simulink model "Ford_T3T6_ArchCnctnDigrm"  (R2016b)
settings: Solver=FixedStepDiscrete  StartTime=0.0  StopTime=10.0  RelTol=1e-3  EnableMultiTasking=on
libraries: canmsglib x15
(part 3 of 15)

== system Ford_T3T6_ArchCnctnDigrm/States and Modes ==
  note: Use Ground if we are using only Gate drive 0 control
  note: T3 does not use SF061
      | (SteerMod)
  note: ASIL D
  note: ASIL D
  note: ASIL D
  note: NM001
  note: NM001
  note: ASIL D
  ES002A_McuDiagc : Subsystem  Tag=3.0.1  Description=This FDD contains uCDiagnostics that are implemented purely with software and are not dependent upon electrical architecture.
      settings: AttributesFormatString=Version: %<Tag>
  ES100A_SysStMod : Subsystem  Tag=1.3.0  Description=Controls the operating state of the system
      settings: AttributesFormatString=Version: %<Tag>
  Ground : Ground
  SF048A_TqLoa : Subsystem  Tag=1.4.1  Description=This function provides a position-based assist command. It also outputs a validity flag to indicate if the TrqLOACmd is valid.
      settings: AttributesFormatString=Version: %<Tag>
  SF049B_LoaMgr : Subsystem  Tag=1.0.0  Description="This function monitors monitors sensor redundancy and allows the choice of system response to varying numbers and types of sensors being unavailable.  It outputs operating state information that other functions use to modify their own behavior when appropriate.  It also outputs a desired system scale factor and slew rate, arbitrated in SF005A State Output Control and then applied in SF004B Assist Sum and Limit."
      settings: AttributesFormatString=Version: %<Tag>
  SystemStartUpState : Subsystem
  tag scope: HwTqLoaMtgtnEna=global, LoaRateLim=global, LoaSca=global, LoaSt=global, LoopCntr2MilliSec=global, MotAgLoaMtgtnEna=global, MotAndThermProtnLoaMod=global, MotCtrlFastLoopCntr=global, MotCtrlSlowLoopCntr=global, SysSt=global, TqLoaAvl=global, TqLoaCmd=global
  wires:
  ES100A_SysStMod/1(SysSt) -> SystemStartUpState/1(SysSt), [SysSt]
  SystemStartUpState/1(SysStWrmIninCmpl) -> ES100A_SysStMod/6(SysStWrmIninCmpl)
  SystemStartUpState/2(StrtUpSt) -> ES100A_SysStMod/7(StrtUpSt)
  [SysStFltOutpReqDi] -> ES100A_SysStMod/2(SysStFltOutpReqDi)
  [SysStImdtTranReqOff] -> ES100A_SysStMod/3(SysStImdtTranReqOff)
  [SysStReqDi] -> ES100A_SysStMod/4(SysStReqDi)
  [FordSysStReqEna] -> ES100A_SysStMod/5(SysStReqEna)
  [FordPwrSplyEnaReq] -> ES100A_SysStMod/1(PwrSplyEnaReq)
  [CurrMeasIdptSig] -> SF049B_LoaMgr/1(CurrMeasIdptSig)
  [DiagcStsIvtr1Inactv] -> SF049B_LoaMgr/2(DiagcStsIvtr1Inactv)
  [DiagcStsIvtr2Inactv] -> SF049B_LoaMgr/3(DiagcStsIvtr2Inactv)
  [HwTqIdptSig] -> SF049B_LoaMgr/4(HwTqIdptSig)
  [IvtrFetFltTyp] -> SF049B_LoaMgr/5(IvtrFetFltTyp)
  [LoaScaDi] -> SF049B_LoaMgr/6(LoaScaDi)
  [MotAgMeclIdptSig] -> SF049B_LoaMgr/7(MotAgMeclIdptSig)
  [MotAgSnsrlsAvl] -> SF049B_LoaMgr/8(MotAgSnsrlsAvl)
  [TqLoaAvl] -> SF049B_LoaMgr/9(TqLoaAvl)
  Ground/1 -> SF049B_LoaMgr/10(VehSteerMod)
  [SetNtcSts10] -> SF049B_LoaMgr/11(SetNtcSts)
  SF049B_LoaMgr/1(HwTqLoaMtgtnEna) -> [HwTqLoaMtgtnEna]
  SF049B_LoaMgr/2(LoaRateLim) -> [LoaRateLim]
  SF049B_LoaMgr/3(LoaSca) -> [LoaSca]
  SF049B_LoaMgr/4(LoaSt) -> [LoaSt]
  SF049B_LoaMgr/5(MotAgLoaMtgtnEna) -> [MotAgLoaMtgtnEna]
  SF049B_LoaMgr/6(MotAndThermProtnLoaMod) -> [MotAndThermProtnLoaMod]
  [MotAgLoaMtgtnEna] -> SF048A_TqLoa/1(MotAgLoaMtgtnEna)
  [MotVelCrf] -> SF048A_TqLoa/2(MotVelCrf)
  [PinionAgArbn] -> SF048A_TqLoa/3(PinionAg)
  [PinionAgConf] -> SF048A_TqLoa/4(PinionAgConf)
  [VehLatA] -> SF048A_TqLoa/5(VehLatA)
  [VehLatAVld] -> SF048A_TqLoa/6(VehLatAVld)
  [VehSpd] -> SF048A_TqLoa/7(VehSpd)
  [VehSpdVld] -> SF048A_TqLoa/8(VehSpdVld)
  SF048A_TqLoa/1(TqLoaAvl) -> [TqLoaAvl]
  SF048A_TqLoa/2(TqLoaCmd) -> [TqLoaCmd]
  [FastLoopCntr] -> ES002A_McuDiagc/1(FastLoopCntr)
  [SlowLoopCntr] -> ES002A_McuDiagc/2(SlowLoopCntr)
  [SysSt] -> ES002A_McuDiagc/3(SysSt)
  [MotCtrlLoopCntr2MilliSec] -> ES002A_McuDiagc/4(MotCtrlLoopCntr2MilliSec)
  [ReadErrInjReg] -> ES002A_McuDiagc/5(ReadErrInjReg)
  [SetNtcSts10] -> ES002A_McuDiagc/6(SetNtcSts)
  [StrtErrInjCntr] -> ES002A_McuDiagc/7(StrtErrInjCntr)
  ES002A_McuDiagc/1(LoopCntr2MilliSec) -> [LoopCntr2MilliSec]
  ES002A_McuDiagc/2(MotCtrlFastLoopCntr) -> [MotCtrlFastLoopCntr]
  ES002A_McuDiagc/3(MotCtrlSlowLoopCntr) -> [MotCtrlSlowLoopCntr]

== system Ford_T3T6_ArchCnctnDigrm/Support Functions ==
  note: ASIL D
  AR100A_NxtrMath : Subsystem  Tag=1.1.0  Description="The Nexteer math encompasses a number of inline functions for use in other software components.  In addition, it contains the functionality for setting a trouble code when an error is detected by the C standard library."
      settings: AttributesFormatString=Version: %<Tag>
  AR200A_NxtrSuprt : Subsystem  Tag=1.0.0
      settings: AttributesFormatString=Version: %<Tag>
  AR999A_ArchGlbPrm : Subsystem  Tag=1.3.0  Description="The ArchGlbPrm component contains global constants that are either \"mathematical\" (e.g. the value of pi) or software-oriented (e.g. the value to be used as the zero threshold for float32 comparisons) in nature.  The constants are defined in AR999A_ArchGlbPrm_DataDict.m and implemented as #define statements in \"ArchGlbPrm.h\"."
      settings: AttributesFormatString=Version: %<Tag>
  ES101AProxy10_DiagcMgrProxy10 : Subsystem  Tag=5.3.X  Description="This function is responsible for storing NTC Information, clearing NTCs on a periodic basis and providing an interface to access DiagcMgr to other components in each application. This is accomplished by having a copy of this component in each of the appication. The \"X\" that is being used across the function signifies the which appication it belongs to. This is a generic copy and this copy shall be duplicated in each application with \"X\" being replaced by the application number."
      settings: AttributesFormatString=Version: %<Tag>
  ES101AProxy6_DiagcMgrProxy6 : Subsystem  Tag=5.3.X  Description="This function is responsible for storing NTC Information, clearing NTCs on a periodic basis and providing an interface to access DiagcMgr to other components in each application. This is accomplished by having a copy of this component in each of the appication. The \"X\" that is being used across the function signifies the which appication it belongs to. This is a generic copy and this copy shall be duplicated in each application with \"X\" being replaced by the application number."
      settings: AttributesFormatString=Version: %<Tag>
  ES101AProxy7_DiagcMgrProxy7 : Subsystem  Tag=5.3.X  Description="This function is responsible for storing NTC Information, clearing NTCs on a periodic basis and providing an interface to access DiagcMgr to other components in each application. This is accomplished by having a copy of this component in each of the appication. The \"X\" that is being used across the function signifies the which appication it belongs to. This is a generic copy and this copy shall be duplicated in each application with \"X\" being replaced by the application number."
      settings: AttributesFormatString=Version: %<Tag>
  ES101AProxy8_DiagcMgrProxy8 : Subsystem  Tag=5.3.X  Description="This function is responsible for storing NTC Information, clearing NTCs on a periodic basis and providing an interface to access DiagcMgr to other components in each application. This is accomplished by having a copy of this component in each of the appication. The \"X\" that is being used across the function signifies the which appication it belongs to. This is a generic copy and this copy shall be duplicated in each application with \"X\" being replaced by the application number."
      settings: AttributesFormatString=Version: %<Tag>
  ES101AProxy9_DiagcMgrProxy9 : Subsystem  Tag=5.3.X  Description="This function is responsible for storing NTC Information, clearing NTCs on a periodic basis and providing an interface to access DiagcMgr to other components in each application. This is accomplished by having a copy of this component in each of the appication. The \"X\" that is being used across the function signifies the which appication it belongs to. This is a generic copy and this copy shall be duplicated in each application with \"X\" being replaced by the application number."
      settings: AttributesFormatString=Version: %<Tag>
  ES999A_ElecGlbPrm : Subsystem  Tag=6.7.0  Description=Electrical Global Parameters
      settings: AttributesFormatString=Version: %<Tag>
  SF999A_SysGlbPrm : Subsystem  Tag=1.4.0  Description=SF999A is a global collection of calibrations and constants that commonly get shared across software components.
      settings: AttributesFormatString=Version: %<Tag>
  tag scope: GetDiagcDataAppl10=global, GetDiagcDataAppl6=global, GetDiagcDataAppl7=global, GetDiagcDataAppl8=global, GetDiagcDataAppl9=global, GetNtcActv10=global, GetNtcActv6=global, GetNtcActv7=global, GetNtcActv8=global, GetNtcActv9=global, GetNtcDebCntrAppl10=global, GetNtcDebCntrAppl6=global, GetNtcDebCntrAppl7=global, GetNtcDebCntrAppl8=global, GetNtcDebCntrAppl9=global, GetNtcInfoAppl10=global, GetNtcInfoAppl6=global, GetNtcInfoAppl7=global, GetNtcInfoAppl8=global, GetNtcInfoAppl9=global, GetNtcQlfrSts10=global, GetNtcQlfrSts6=global, GetNtcQlfrSts7=global, GetNtcQlfrSts8=global, GetNtcQlfrSts9=global, GetNtcSts10=global, GetNtcSts6=global, GetNtcSts7=global, GetNtcSts8=global, GetNtcSts9=global, InjSwFpuErr=global, SetNtcSts10=global, SetNtcSts6=global, SetNtcSts7=global, SetNtcSts8=global, SetNtcSts9=global, SetNtcStsAndSnpshtData10=global, SetNtcStsAndSnpshtData6=global, SetNtcStsAndSnpshtData7=global, SetNtcStsAndSnpshtData8=global, SetNtcStsAndSnpshtData9=global, gh_set_errno=global
  wires:
  [ReadErrInjReg] -> AR100A_NxtrMath/1(ReadErrInjReg)
  [SetNtcSts10] -> AR100A_NxtrMath/2(SetNtcSts)
  AR100A_NxtrMath/1(InjSwFpuErr) -> [InjSwFpuErr]
  AR100A_NxtrMath/2(gh_set_errno) -> [gh_set_errno]
  [ClrDiagcFlgProxy] -> ES101AProxy10_DiagcMgrProxy10/1(ClrDiagcFlgProxy)
  [DiagcMgrIninCore] -> ES101AProxy10_DiagcMgrProxy10/2(DiagcMgrIninCore)
  [GetNtcActvCore] -> ES101AProxy10_DiagcMgrProxy10/3(GetNtcActvCore)
  [GetNtcQlfrStsCore] -> ES101AProxy10_DiagcMgrProxy10/4(GetNtcQlfrStsCore)
  [GetNtcStsCore] -> ES101AProxy10_DiagcMgrProxy10/5(GetNtcStsCore)
  [SetNtcStsCore] -> ES101AProxy10_DiagcMgrProxy10/6(SetNtcStsCore)
  ES101AProxy10_DiagcMgrProxy10/1(GetDiagcDataAppl10) -> [GetDiagcDataAppl10]
  ES101AProxy10_DiagcMgrProxy10/2(GetNtcActv10) -> [GetNtcActv10]
  ES101AProxy10_DiagcMgrProxy10/3(GetNtcDebCntrAppl10) -> [GetNtcDebCntrAppl10]
  ES101AProxy10_DiagcMgrProxy10/4(GetNtcInfoAppl10) -> [GetNtcInfoAppl10]
  ES101AProxy10_DiagcMgrProxy10/5(GetNtcQlfrSts10) -> [GetNtcQlfrSts10]
  ES101AProxy10_DiagcMgrProxy10/6(GetNtcSts10) -> [GetNtcSts10]
  ES101AProxy10_DiagcMgrProxy10/7(SetNtcSts10) -> [SetNtcSts10]
  ES101AProxy10_DiagcMgrProxy10/8(SetNtcStsAndSnpshtData10) -> [SetNtcStsAndSnpshtData10]
  [ClrDiagcFlgProxy] -> ES101AProxy8_DiagcMgrProxy8/1(ClrDiagcFlgProxy)
  [DiagcMgrIninCore] -> ES101AProxy8_DiagcMgrProxy8/2(DiagcMgrIninCore)
  [GetNtcActvCore] -> ES101AProxy8_DiagcMgrProxy8/3(GetNtcActvCore)
  [GetNtcQlfrStsCore] -> ES101AProxy8_DiagcMgrProxy8/4(GetNtcQlfrStsCore)
  [GetNtcStsCore] -> ES101AProxy8_DiagcMgrProxy8/5(GetNtcStsCore)
  [SetNtcStsCore] -> ES101AProxy8_DiagcMgrProxy8/6(SetNtcStsCore)
  ES101AProxy8_DiagcMgrProxy8/1(GetDiagcDataAppl8) -> [GetDiagcDataAppl8]
  ES101AProxy8_DiagcMgrProxy8/2(GetNtcActv8) -> [GetNtcActv8]
  ES101AProxy8_DiagcMgrProxy8/3(GetNtcDebCntrAppl8) -> [GetNtcDebCntrAppl8]
  ES101AProxy8_DiagcMgrProxy8/4(GetNtcInfoAppl8) -> [GetNtcInfoAppl8]
  ES101AProxy8_DiagcMgrProxy8/5(GetNtcQlfrSts8) -> [GetNtcQlfrSts8]
  ES101AProxy8_DiagcMgrProxy8/6(GetNtcSts8) -> [GetNtcSts8]
  ES101AProxy8_DiagcMgrProxy8/7(SetNtcSts8) -> [SetNtcSts8]
  ES101AProxy8_DiagcMgrProxy8/8(SetNtcStsAndSnpshtData8) -> [SetNtcStsAndSnpshtData8]
  [ClrDiagcFlgProxy] -> ES101AProxy6_DiagcMgrProxy6/1(ClrDiagcFlgProxy)
  [DiagcMgrIninCore] -> ES101AProxy6_DiagcMgrProxy6/2(DiagcMgrIninCore)
  [GetNtcActvCore] -> ES101AProxy6_DiagcMgrProxy6/3(GetNtcActvCore)
  [GetNtcQlfrStsCore] -> ES101AProxy6_DiagcMgrProxy6/4(GetNtcQlfrStsCore)
  [GetNtcStsCore] -> ES101AProxy6_DiagcMgrProxy6/5(GetNtcStsCore)
  [SetNtcStsCore] -> ES101AProxy6_DiagcMgrProxy6/6(SetNtcStsCore)
  ES101AProxy6_DiagcMgrProxy6/1(GetDiagcDataAppl6) -> [GetDiagcDataAppl6]
  ES101AProxy6_DiagcMgrProxy6/2(GetNtcActv6) -> [GetNtcActv6]
  ES101AProxy6_DiagcMgrProxy6/3(GetNtcDebCntrAppl6) -> [GetNtcDebCntrAppl6]
  ES101AProxy6_DiagcMgrProxy6/4(GetNtcInfoAppl6) -> [GetNtcInfoAppl6]
  ES101AProxy6_DiagcMgrProxy6/5(GetNtcQlfrSts6) -> [GetNtcQlfrSts6]
  ES101AProxy6_DiagcMgrProxy6/6(GetNtcSts6) -> [GetNtcSts6]
  ES101AProxy6_DiagcMgrProxy6/7(SetNtcSts6) -> [SetNtcSts6]
  ES101AProxy6_DiagcMgrProxy6/8(SetNtcStsAndSnpshtData6) -> [SetNtcStsAndSnpshtData6]
  [ClrDiagcFlgProxy] -> ES101AProxy7_DiagcMgrProxy7/1(ClrDiagcFlgProxy)
  [DiagcMgrIninCore] -> ES101AProxy7_DiagcMgrProxy7/2(DiagcMgrIninCore)
  [GetNtcActvCore] -> ES101AProxy7_DiagcMgrProxy7/3(GetNtcActvCore)
  [GetNtcQlfrStsCore] -> ES101AProxy7_DiagcMgrProxy7/4(GetNtcQlfrStsCore)
  [GetNtcStsCore] -> ES101AProxy7_DiagcMgrProxy7/5(GetNtcStsCore)
  [SetNtcStsCore] -> ES101AProxy7_DiagcMgrProxy7/6(SetNtcStsCore)
  ES101AProxy7_DiagcMgrProxy7/1(GetDiagcDataAppl7) -> [GetDiagcDataAppl7]
  ES101AProxy7_DiagcMgrProxy7/2(GetNtcActv7) -> [GetNtcActv7]
  ES101AProxy7_DiagcMgrProxy7/3(GetNtcDebCntrAppl7) -> [GetNtcDebCntrAppl7]
  ES101AProxy7_DiagcMgrProxy7/4(GetNtcInfoAppl7) -> [GetNtcInfoAppl7]
  ES101AProxy7_DiagcMgrProxy7/5(GetNtcQlfrSts7) -> [GetNtcQlfrSts7]
  ES101AProxy7_DiagcMgrProxy7/6(GetNtcSts7) -> [GetNtcSts7]
  ES101AProxy7_DiagcMgrProxy7/7(SetNtcSts7) -> [SetNtcSts7]
  ES101AProxy7_DiagcMgrProxy7/8(SetNtcStsAndSnpshtData7) -> [SetNtcStsAndSnpshtData7]
  [ClrDiagcFlgProxy] -> ES101AProxy9_DiagcMgrProxy9/1(ClrDiagcFlgProxy)
  [DiagcMgrIninCore] -> ES101AProxy9_DiagcMgrProxy9/2(DiagcMgrIninCore)
  [GetNtcActvCore] -> ES101AProxy9_DiagcMgrProxy9/3(GetNtcActvCore)
  [GetNtcQlfrStsCore] -> ES101AProxy9_DiagcMgrProxy9/4(GetNtcQlfrStsCore)
  [GetNtcStsCore] -> ES101AProxy9_DiagcMgrProxy9/5(GetNtcStsCore)
  [SetNtcStsCore] -> ES101AProxy9_DiagcMgrProxy9/6(SetNtcStsCore)
  ES101AProxy9_DiagcMgrProxy9/1(GetDiagcDataAppl9) -> [GetDiagcDataAppl9]
  ES101AProxy9_DiagcMgrProxy9/2(GetNtcActv9) -> [GetNtcActv9]
  ES101AProxy9_DiagcMgrProxy9/3(GetNtcDebCntrAppl9) -> [GetNtcDebCntrAppl9]
  ES101AProxy9_DiagcMgrProxy9/4(GetNtcInfoAppl9) -> [GetNtcInfoAppl9]
  ES101AProxy9_DiagcMgrProxy9/5(GetNtcQlfrSts9) -> [GetNtcQlfrSts9]
  ES101AProxy9_DiagcMgrProxy9/6(GetNtcSts9) -> [GetNtcSts9]
  ES101AProxy9_DiagcMgrProxy9/7(SetNtcSts9) -> [SetNtcSts9]
  ES101AProxy9_DiagcMgrProxy9/8(SetNtcStsAndSnpshtData9) -> [SetNtcStsAndSnpshtData9]

== system Ford_T3T6_ArchCnctnDigrm/System Diagnostic Action ==
  note: NM001
  note: Diag Manager Stub
  note: ASIL D
  note: ASIL D
  note: Diag Manager Stub
  note: NM001
  note: NM001
  note: NM001
  ES101ACore_DiagcMgr : Subsystem  Tag=5.2.X  Description=This function is responsible for handling all the NTCs that are used by different FDDs. The Diagnostic Manager sets the NTC called by any component and requests the system to either ramp down to Disable or take no action
      settings: AttributesFormatString=Version: %<Tag>
  Ground{,1..3} (4 alike) : Ground
  SF005A_StOutpCtrl : Subsystem  Tag=1.4.1  Description="The State Output Control Function implements the system ramping functions based on inputs from other modules.  Ramping due to diagnostics and other functions are requested and this function does the actual implementation of the ramping.  The ramping rate can also be increased through the use of a serial comm service."
      settings: AttributesFormatString=Version: %<Tag>
  Terminator : Terminator
  tag scope: ClrAllDiagc=global, ClrDiagcFlgProxy=global, ClrLtchCntrData=global, ClrSnpshtData=global, CnvSnpshtData_f32=global, CnvSnpshtData_logl=global, CnvSnpshtData_s08=global, CnvSnpshtData_s16=global, CnvSnpshtData_s32=global, CnvSnpshtData_u08=global, CnvSnpshtData_u16=global, DiagcMgrIninCore=global, DiagcMgrPwrDwn=global, DiagcStsCtrldShtDwnFltPrsnt=global, GetNtcActvCore=global, GetNtcQlfrStsCore=global, GetNtcStsCore=global, ReadLtchCntrData=global, ReadNtcFltAry=global, ReadNtcInfoAndDebCntr=global, ReadSnpshtData=global, RestoreDiagcMgrLtchCntrAryDft=global, RestoreNtcFltAryDft=global, RestoreSnpshtAryDft=global, SetNtcStsCore=global, SysMotTqCmdSca=global, SysStFltOutpReqDi=global, SysStReqDi=global, UpdDtcEnaCdn=global
  wires:
  SF005A_StOutpCtrl/1(SysMotTqCmdSca) -> [SysMotTqCmdSca]
  [LoaRateLim] -> SF005A_StOutpCtrl/2(LoaRateLim)
  [LoaSca] -> SF005A_StOutpCtrl/3(LoaSca)
  [SysMotTqCmdRampRateDi] -> SF005A_StOutpCtrl/7(SysMotTqCmdRampRateDi)
  Ground3/1 -> SF005A_StOutpCtrl/8(SysOperMotTqCmdSca)
  Ground2/1 -> SF005A_StOutpCtrl/9(SysOperRampRate)
  SF005A_StOutpCtrl/2(SysStReqDi) -> [SysStReqDi]
  [MotTqTranlDampgCmpl] -> SF005A_StOutpCtrl/4(MotTqTranlDampgCmpl)
  [HwTq] -> ES101ACore_DiagcMgr/3(HwTq)
  [EcuTFild] -> ES101ACore_DiagcMgr/2(EcuTFild)
  [IgnCntr] -> ES101ACore_DiagcMgr/4(IgnCntr)
  [BrdgVltg] -> ES101ACore_DiagcMgr/1(BrdgVltg)
  [MfgDiagcInhb] -> ES101ACore_DiagcMgr/5(MfgDiagcInhb)
  [MfgEnaSt] -> ES101ACore_DiagcMgr/6(MfgEnaSt)
  [MotTqCmdPwrLimd] -> ES101ACore_DiagcMgr/7(MotTqCmdMrfScad)
  [SysSt] -> ES101ACore_DiagcMgr/9(SysSt)
  [SwApplCrc] -> ES101ACore_DiagcMgr/8(SwApplCrc)
  [Dem_GetDTCOfEvent] -> ES101ACore_DiagcMgr/11(Dem_GetDTCOfEvent)
  [Dem_ClearDTC] -> ES101ACore_DiagcMgr/10(Dem_ClearDTC)
  [GetDiagcDataApplX] -> ES101ACore_DiagcMgr/16(GetDiagcDataApplX)
  [Dem_SetEventStatus] -> ES101ACore_DiagcMgr/12(Dem_SetEventStatus)
  [NvMProxy_SetRamBlockStatus] -> ES101ACore_DiagcMgr/15(DiagcMgrNtcFltAry_SetRamBlockStatus)
  [NvMProxy_SetRamBlockStatus] -> ES101ACore_DiagcMgr/13(DiagcMgrApplCrc_SetRamBlockStatus)
  [NvMProxy_SetRamBlockStatus] -> ES101ACore_DiagcMgr/14(DiagcMgrLtchCntrAry_SetRamBlockStatus)
  [GetMcuDiagcSpplData] -> ES101ACore_DiagcMgr/17(GetMcuDiagcSpplData)
  [GetNtcDebCntrApplX] -> ES101ACore_DiagcMgr/18(GetNtcDebCntrApplX)
  [NvMProxy_SetRamBlockStatus] -> ES101ACore_DiagcMgr/20(SnpshtDataAry_SetRamBlockStatus)
  [GetNtcInfoApplX] -> ES101ACore_DiagcMgr/19(GetNtcInfoApplX)
  ES101ACore_DiagcMgr/27(RestoreNtcFltAryDft) -> [RestoreNtcFltAryDft]
  ES101ACore_DiagcMgr/28(RestoreSnpshtAryDft) -> [RestoreSnpshtAryDft]
  ES101ACore_DiagcMgr/29(SetNtcStsCore) -> [SetNtcStsCore]
  ES101ACore_DiagcMgr/30(UpdDtcEnaCdn) -> [UpdDtcEnaCdn]
  ES101ACore_DiagcMgr/1(ClrDiagcFlgProxy) -> [ClrDiagcFlgProxy]
  ES101ACore_DiagcMgr/2(DiagcStsCtrldShtDwnFltPrsnt) -> [DiagcStsCtrldShtDwnFltPrsnt]
  ES101ACore_DiagcMgr/7(ClrAllDiagc) -> [ClrAllDiagc]
  ES101ACore_DiagcMgr/9(ClrSnpshtData) -> [ClrSnpshtData]
  ES101ACore_DiagcMgr/21(GetNtcStsCore) -> [GetNtcStsCore]
  ES101ACore_DiagcMgr/20(GetNtcQlfrStsCore) -> [GetNtcQlfrStsCore]
  ES101ACore_DiagcMgr/19(GetNtcActvCore) -> [GetNtcActvCore]
  ES101ACore_DiagcMgr/18(DiagcMgrPwrDwn) -> [DiagcMgrPwrDwn]
  ES101ACore_DiagcMgr/17(DiagcMgrIninCore) -> [DiagcMgrIninCore]
  ES101ACore_DiagcMgr/25(ReadSnpshtData) -> [ReadSnpshtData]
  ES101ACore_DiagcMgr/24(ReadNtcInfoAndDebCntr) -> [ReadNtcInfoAndDebCntr]
  ES101ACore_DiagcMgr/23(ReadNtcFltAry) -> [ReadNtcFltAry]
  ES101ACore_DiagcMgr/26(RestoreDiagcMgrLtchCntrAryDft) -> [RestoreDiagcMgrLtchCntrAryDft]
  ES101ACore_DiagcMgr/22(ReadLtchCntrData) -> [ReadLtchCntrData]
  ES101ACore_DiagcMgr/8(ClrLtchCntrData) -> [ClrLtchCntrData]
  ES101ACore_DiagcMgr/4(SysDiMotTqCmdSca) -> SF005A_StOutpCtrl/5(SysDiMotTqCmdSca)
  ES101ACore_DiagcMgr/5(SysDiRampRate) -> SF005A_StOutpCtrl/6(SysDiRampRate)
  ES101ACore_DiagcMgr/6(SysStFltOutpReqDi) -> [SysStFltOutpReqDi]
  ES101ACore_DiagcMgr/3(DiagcStsNonRcvrlReqDiFltPrsnt) -> Terminator/1
  Ground/1 -> SF005A_StOutpCtrl/12(VehStrtStopRampRate)
  Ground1/1 -> SF005A_StOutpCtrl/11(VehStrtStopMotTqCmdSca)
  [DiagcStsCtrldShtDwnFltPrsnt] -> SF005A_StOutpCtrl/1(DiagcStsCtrldShtDwnFltPrsnt)
  [SysStFltOutpReqDi] -> SF005A_StOutpCtrl/10(SysStFltOutpReqDi)
  ES101ACore_DiagcMgr/10(CnvSnpshtData_f32) -> [CnvSnpshtData_f32]
  ES101ACore_DiagcMgr/11(CnvSnpshtData_logl) -> [CnvSnpshtData_logl]
  ES101ACore_DiagcMgr/12(CnvSnpshtData_s08) -> [CnvSnpshtData_s08]
  ES101ACore_DiagcMgr/13(CnvSnpshtData_s16) -> [CnvSnpshtData_s16]
  ES101ACore_DiagcMgr/14(CnvSnpshtData_s32) -> [CnvSnpshtData_s32]
  ES101ACore_DiagcMgr/15(CnvSnpshtData_u08) -> [CnvSnpshtData_u08]
  ES101ACore_DiagcMgr/16(CnvSnpshtData_u16) -> [CnvSnpshtData_u16]

== system Ford_T3T6_ArchCnctnDigrm/System Wellness ==
  note: ASIL D Safety Mech
  CM111A_VrfyCritReg : Subsystem  Tag=4.1.0  Description=This component describes the functions which verify critical registers.
      settings: AttributesFormatString=Version: %<Tag>
  SF058B_SysOutpPrsntCpby : Subsystem  Tag=1.1.0  Description=This function uses motor envelope to estimate the maximum motor torque available at the present time,maximum handwheel velocity, and the factors that limiting the maximum handwheel velocity(e.g. thermal limit, voltage, friction, and system status that is dual controller v.s. single controller).
      settings: AttributesFormatString=Version: %<Tag>
  tag scope: EcuStsFlg=global, FricFlg=global, InjVrfyCritRegErr=global, MCalReadVrfyFailFltInfo=global, MaxHwVel=global, MotKneePtTq=global, MotKneePtVel=global, MotTqAvl=global, MotZeroPtVel=global, ThermFlg=global, ThermFlgCombd=global, VltgFlg=global, VltgFlgCombd=global
  wires:
  [ClrErrInjReg] -> CM111A_VrfyCritReg/1(ClrErrInjReg)
  [MCalWrVrfyRegFltInfoStorg_GetErrorStatus] -> CM111A_VrfyCritReg/2(MCalWrVrfyRegFltInfoStorg_GetErrorStatus)
  [MCalWrVrfyRegFltInfoStorg_SetRamBlockStatus] -> CM111A_VrfyCritReg/3(MCalWrVrfyRegFltInfoStorg_SetRamBlockStatus)
  [ReadErrInjReg] -> CM111A_VrfyCritReg/4(ReadErrInjReg)
  [SetNtcSts9] -> CM111A_VrfyCritReg/5(SetNtcSts)
  CM111A_VrfyCritReg/1(InjVrfyCritRegErr) -> [InjVrfyCritRegErr]
  CM111A_VrfyCritReg/2(MCalReadVrfyFailFltInfo) -> [MCalReadVrfyFailFltInfo]
  [BrdgVltg] -> SF058B_SysOutpPrsntCpby/1(BrdgVltg)
  [ImcSysSt] -> SF058B_SysOutpPrsntCpby/2(ImcSysSt)
  [ImcSysStVld] -> SF058B_SysOutpPrsntCpby/3(ImcSysStVld)
  [MotBackEmfConEstimd] -> SF058B_SysOutpPrsntCpby/4(MotBackEmfConEstimd)
  [MotVelCrf] -> SF058B_SysOutpPrsntCpby/5(MotVelCrf)
  [SysFricEstimd] -> SF058B_SysOutpPrsntCpby/6(SysFricEstimd)
  [SysSt] -> SF058B_SysOutpPrsntCpby/7(SysSt)
  [ThermMotTqLimCdnd] -> SF058B_SysOutpPrsntCpby/8(ThermMotTqLimCdnd)
  [VehSpd] -> SF058B_SysOutpPrsntCpby/9(VehSpd)
  [GetSigImcData_f32] -> SF058B_SysOutpPrsntCpby/10(GetSigImcData_f32)
  [GetSigImcData_logl] -> SF058B_SysOutpPrsntCpby/11(GetSigImcData_logl)
  SF058B_SysOutpPrsntCpby/1(EcuStsFlg) -> [EcuStsFlg]
  SF058B_SysOutpPrsntCpby/2(FricFlg) -> [FricFlg]
  SF058B_SysOutpPrsntCpby/3(MaxHwVel) -> [MaxHwVel]
  SF058B_SysOutpPrsntCpby/4(MotKneePtTq) -> [MotKneePtTq]
  SF058B_SysOutpPrsntCpby/5(MotKneePtVel) -> [MotKneePtVel]
  SF058B_SysOutpPrsntCpby/6(MotTqAvl) -> [MotTqAvl]
  SF058B_SysOutpPrsntCpby/7(MotZeroPtVel) -> [MotZeroPtVel]
  SF058B_SysOutpPrsntCpby/8(ThermFlg) -> [ThermFlg]
  SF058B_SysOutpPrsntCpby/9(ThermFlgCombd) -> [ThermFlgCombd]
  SF058B_SysOutpPrsntCpby/10(VltgFlg) -> [VltgFlg]
  SF058B_SysOutpPrsntCpby/11(VltgFlgCombd) -> [VltgFlgCombd]

== system Ford_T3T6_ArchCnctnDigrm/Vector Components Base Software ==
  AR001ADio_Dio : Subsystem  Tag=0.0.X  Description=The DIO Driver provides services for reading and writing to/from: DIO Channels (Pins), DIO Ports, DIO Channel Groups. The behaviour of those services is synchronous. This module works on pins and ports which are configured by the PORT driver for this purpose. For this reason, there is no configuration and initialization of this port structure in the DIO Driver.
      settings: AttributesFormatString=Version: %<Tag>
  AR001AEcuM_EcuM : Subsystem  Tag=0.0.X  Description=The ECU Manager module (as specified in this document) is a basic software module (see [1]) that manages common aspects of ECU states. Specifically, the ECU Manager module -Initializes and de-initializes the OS, the SchM and the BswM as well as some basic software driver modules. - configures the ECU for SLEEP and SHUTDOWN when requested. - manages all wakeup events on the ECU. The ECU Manager module provides the wakeup validation protocol to distinguish ï¿½realï¿½ wakeup events from ï¿½erraticï¿½ ones.
      settings: AttributesFormatString=Version: %<Tag>
  AR001AFls_Fls : Subsystem  Tag=0.0.X  Description=The flash driver provides services for reading, writing and erasing flash memory and a configuration interface for setting / resetting the write / erase protection if supported by the underlying hardware. In application mode of the ECU, the flash driver is only to be used by the Flash EEPROM emulation module for writing data. It is not intended to write program code to flash memory in application mode. This shall be done in boot mode which is out of scope of AUTOSAR.
      settings: AttributesFormatString=Version: %<Tag>
  AR001APort_Port : Subsystem  Tag=0.0.X  Description=This driver specification is applicable for on-chip ports and port pins. This module shall provide the service for initializing the whole PORT structure of the microcontroller. Many ports and port pins can be assigned to various functionalities, e.g. General purpose I/O, ADC, SPI, SCI, PWM, CAN, LIN, etc. For this reason, there shall be an overall configuration and initialization of this port structure. The configuration and mode of these port pins is microcontroller and ECU dependent. Port initialisation data shall be written to each port as efficiently as possible. This PORT driver module shall complete the overall configuration and initialisation of the port structure which is used in the DIO driver module. Therefore, the DIO driver works on pins and ports which are configured by the PORT driver. The PORT driver shall be initialised prior to use of the DIO functions. Otherwise DIO functions will exhibit undefined behaviour.
      settings: AttributesFormatString=Version: %<Tag>
  AR001ASpi_Spi : Subsystem  Tag=0.0.X  Description=The SPI Handler/Driver provides services for reading from and writing to devices connected via SPI busses. It provides access to SPI communication to several users (e.g. EEPROM, Watchdog, I/O ASICs). It also provides the required mechanism to configure the onchip SPI peripheral.
      settings: AttributesFormatString=Version: %<Tag>
  CAN : Subsystem
  COM : Subsystem
  DIAG : Subsystem
  IO : Subsystem
  MCAL : Subsystem
  MEM : Subsystem
  OS : Subsystem
  SYS : Subsystem
  tag scope: Spi_AsyncTransmit=global, Spi_GetSequenceResult=global, Spi_ReadIB=global, Spi_WriteIB=global
  wires:
  AR001ASpi_Spi/1(Spi_AsyncTransmit) -> [Spi_AsyncTransmit]
  AR001ASpi_Spi/2(Spi_GetSequenceResult) -> [Spi_GetSequenceResult]
  AR001ASpi_Spi/3(Spi_ReadIB) -> [Spi_ReadIB]
  AR001ASpi_Spi/4(Spi_WriteIB) -> [Spi_WriteIB]

== system Ford_T3T6_ArchCnctnDigrm/Vehicle Com ==
  note: ASIL B
  note: Missing MM082
  note: ASIL B
  note: ASIL B
  note: NM001
  note: NM001
  note: From MM066
  CF049A_FordVehSpdArbn : Subsystem  Tag=1.0.0  Description=This function determines vehicle speed to an ASIL Dlevel.The function contains calculation of vehiclespeed from tire circumference and wheel speed, as well as arbitration of vehicle speeds. The output FordVehicle Speed will feed SF33A
      settings: AttributesFormatString=Version: %<Tag>
  CF100A_FordCanSigVldFlgGenr : Subsystem  Tag=1.0.X  Description="The purpose of the Ford CAN Signal Valid Flag Generator is to generate Ford-In-House valid flags that depend on CAN signals from multiple CAN messages.  This function also takes in those signals and outputs them as a pass-through so that they are in sync with their corresponding valid flags."
      settings: AttributesFormatString=Version: %<Tag>
  Rx Messages : Subsystem
  SF033A_VehSigCdng : Subsystem  Tag=2.3.0  Description=Serial communications signals are received and processed via SER. SER also determines the validity of an incoming signal and may choose to replace the serial comm value with a calibrated default value.
      settings: AttributesFormatString=Version: %<Tag>
  Tx Messages : Subsystem
  tag scope: FordVehActvFrntSteerModlSteerWhlAgRawPassd=global, FordVehActvParkAssiVld=global, FordVehGearLvrPosnPassd=global, FordVehGearLvrPosnVld=global, FordVehGearPosnRawPassd=global, FordVehParkAidModlReqdAgPassd=global, FordVehParkAidModlReqdStsPassd=global, FordVehSpd=global, FordVehSpdLoQly=global, FordVehSpdLoQlyVld=global, FordVehSpdVld=global, FordVehTrlrAgOffsDirRawPassd=global, FordVehTrlrAidIdnNrRawPassd=global, FordVehTrlrAidSetUpRawPassd=global, FordVehTrlrAidTrlrRvsGuidcStsPassd=global, FordVehTrlrBackUpAssiEnaVld=global, FordVehTrlrBackUpAssiRvsVld=global, FordVehTrlrEnaReqRawPassd=global, FordVehTrlrIdnTypRawPassd=global, FordVehTrlrRvsCnclReqRawPassd=global, FordVehTrlrRvsEnaRawPassd=global, FordVehTrlrRvsMsgTxtReqRawPassd=global, FordVehTrsmDesGearRawPassd=global, VehLatA=global, VehLatAEstimd=global, VehLatAEstimdVld=global, VehLatAVld=global, VehLgtA=global, VehLgtAVld=global, VehSpdSigCdnd=global, VehSpdVld=global, VehYawRate=global, VehYawRateVld=global
  wires:
  [HwTq] -> SF033A_VehSigCdng/1(HwTq)
  [FordVehLatACmpd] -> SF033A_VehSigCdng/2(VehLatASerlCom)
  [FordVehLatACmpdVld] -> SF033A_VehSigCdng/3(VehLatAVldSerlCom)
  [FordVehLgtACmpd] -> SF033A_VehSigCdng/4(VehLgtASerlCom)
  [FordVehLgtACmpdVld] -> SF033A_VehSigCdng/5(VehLgtAVldSerlCom)
  [VehSpdOvrd] -> SF033A_VehSigCdng/6(VehSpdOvrd)
  [VehSpdOvrdEna] -> SF033A_VehSigCdng/7(VehSpdOvrdEna)
  [FordVehSpd] -> SF033A_VehSigCdng/8(VehSpdSerlCom)
  [FordVehSpdVld] -> SF033A_VehSigCdng/9(VehSpdVldSerlCom)
  [FordVehYawRateCmpd] -> SF033A_VehSigCdng/10(VehYawRateSerlCom)
  [FordVehYawRateCmpdVld] -> SF033A_VehSigCdng/11(VehYawRateVldSerlCom)
  [FltInj_f32] -> SF033A_VehSigCdng/12(FltInj_f32)
  SF033A_VehSigCdng/1(VehLatA) -> [VehLatA]
  SF033A_VehSigCdng/2(VehLatAEstimd) -> [VehLatAEstimd]
  SF033A_VehSigCdng/3(VehLatAEstimdVld) -> [VehLatAEstimdVld]
  SF033A_VehSigCdng/4(VehLatAVld) -> [VehLatAVld]
  SF033A_VehSigCdng/5(VehLgtA) -> [VehLgtA]
  SF033A_VehSigCdng/6(VehLgtAVld) -> [VehLgtAVld]
  SF033A_VehSigCdng/7(VehSpd) -> [VehSpdSigCdnd]
  SF033A_VehSigCdng/8(VehSpdVld) -> [VehSpdVld]
  SF033A_VehSigCdng/9(VehYawRate) -> [VehYawRate]
  SF033A_VehSigCdng/10(VehYawRateVld) -> [VehYawRateVld]
  [FordAbsPrsnt] -> CF049A_FordVehSpdArbn/1(FordAbsModlPrsnt)
  [FordAbsPrsnt] -> CF049A_FordVehSpdArbn/2(FordEscModlPrsnt)
  [FordVehFrntLeWhlSpd] -> CF049A_FordVehSpdArbn/3(FordVehFrntLeWhlSpd)
  [FordVehFrntLeWhlSpdVld] -> CF049A_FordVehSpdArbn/4(FordVehFrntLeWhlSpdVld)
  [FordVehFrntRiWhlSpd] -> CF049A_FordVehSpdArbn/5(FordVehFrntRiWhlSpd)
  [FordVehFrntRiWhlSpdVld] -> CF049A_FordVehSpdArbn/6(FordVehFrntRiWhlSpdVld)
  [FordVehReLeWhlSpd] -> CF049A_FordVehSpdArbn/7(FordVehReLeWhlSpd)
  [FordVehReLeWhlSpdVld] -> CF049A_FordVehSpdArbn/8(FordVehReLeWhlSpdVld)
  [FordVehReRiWhlSpd] -> CF049A_FordVehSpdArbn/9(FordVehReRiWhlSpd)
  [FordVehReRiWhlSpdVld] -> CF049A_FordVehSpdArbn/10(FordVehReRiWhlSpdVld)
  [FordVehSpdBrkModl] -> CF049A_FordVehSpdArbn/11(FordVehSpdBrkModl)
  [FordVehSpdBrkModlLoQlyVld] -> CF049A_FordVehSpdArbn/12(FordVehSpdBrkModlLoQlyVld)
  [FordVehSpdBrkModlVld] -> CF049A_FordVehSpdArbn/13(FordVehSpdBrkModlVld)
  [FordVehSpdEngModl] -> CF049A_FordVehSpdArbn/14(FordVehSpdEngModl)
  [FordVehSpdEngModlLoQlyVld] -> CF049A_FordVehSpdArbn/15(FordVehSpdEngModlLoQlyVld)
  [FordVehSpdEngModlVld] -> CF049A_FordVehSpdArbn/16(FordVehSpdEngModlVld)
  [NvMProxy_GetErrorStatus] -> CF049A_FordVehSpdArbn/17(FordVehTireCircum_GetErrorStatus)
  CF049A_FordVehSpdArbn/1(FordVehSpd) -> [FordVehSpd]
  CF049A_FordVehSpdArbn/2(FordVehSpdLoQly) -> [FordVehSpdLoQly]
  CF049A_FordVehSpdArbn/3(FordVehSpdLoQlyVld) -> [FordVehSpdLoQlyVld]
  CF049A_FordVehSpdArbn/4(FordVehSpdVld) -> [FordVehSpdVld]
  [FordActvFrntSteerModlSteerWhlAgVldInt] -> CF100A_FordCanSigVldFlgGenr/1(ActvFrntSteerModlSteerWhlAgVldInt)
  [FordVehActvFrntSteerModlSteerWhlAgRaw] -> CF100A_FordCanSigVldFlgGenr/2(FordVehActvFrntSteerModSteerWhlAgRaw)
  [FordVehGearLvrPosn] -> CF100A_FordCanSigVldFlgGenr/3(FordVehGearLvrPosnRaw)
  [FordVehGearPosnRaw] -> CF100A_FordCanSigVldFlgGenr/4(FordVehGearPosnRaw)
  [FordVehParkAidModlReqdAgRaw] -> CF100A_FordCanSigVldFlgGenr/5(FordVehParkAidModlReqdAgRaw)
  [FordVehParkAidModlReqdSts] -> CF100A_FordCanSigVldFlgGenr/6(FordVehParkAidModlReqdStsRaw)
  [FordVehTrlrAgOffsDirRaw] -> CF100A_FordCanSigVldFlgGenr/7(FordVehTrlrAgOffsDirRaw)
  [FordVehTrlrAidIdnNrRaw] -> CF100A_FordCanSigVldFlgGenr/8(FordVehTrlrAidIdnNrRaw)
  [FordVehTrlrAidSetUpRaw] -> CF100A_FordCanSigVldFlgGenr/9(FordVehTrlrAidSetUpRaw)
  [FordVehTrlrAidTrlrRvsGuidcSts] -> CF100A_FordCanSigVldFlgGenr/10(FordVehTrlrAidTrlrRvsGuidcStsRaw)
  [FordVehTrlrEnaReqRaw] -> CF100A_FordCanSigVldFlgGenr/11(FordVehTrlrEnaReqRaw)
  [FordVehTrlrIdnTypRaw] -> CF100A_FordCanSigVldFlgGenr/12(FordVehTrlrIdnTypRaw)
  [FordVehTrlrRvsCnclReqRaw] -> CF100A_FordCanSigVldFlgGenr/13(FordVehTrlrRvsCnclReqRaw)
  [FordVehTrlrRvsEnaRaw] -> CF100A_FordCanSigVldFlgGenr/14(FordVehTrlrRvsEnaRaw)
  [FordVehTrlrRvsMsgTxtReqRaw] -> CF100A_FordCanSigVldFlgGenr/15(FordVehTrlrRvsMsgTxtReqRaw)
  [FordVehTrsmDesGearRaw] -> CF100A_FordCanSigVldFlgGenr/16(FordVehTrsmDesGearRaw)
  [FordVehGearLvrPosnVldInt] -> CF100A_FordCanSigVldFlgGenr/17(GearLvrPosnVldInt)
  [FordVehGearPosnRawVldInt] -> CF100A_FordCanSigVldFlgGenr/18(GearPosnRawVldInt)
  [ImgProcgDataPrsntInt] -> CF100A_FordCanSigVldFlgGenr/19(ImgProcgDataPrsntInt)
  [FordVehParkAidModlReqdAgVldInt] -> CF100A_FordCanSigVldFlgGenr/20(ParkAidModlReqdAgVldInt)
  [FordVehParkAidModlStsVldInt] -> CF100A_FordCanSigVldFlgGenr/21(ParkAidModlReqdStsVldInt)
  [TrlrAidDataPrsntInt] -> CF100A_FordCanSigVldFlgGenr/22(TrlrAidDataPrsntInt)
  [TrlrAidDataThreePrsntInt] -> CF100A_FordCanSigVldFlgGenr/23(TrlrAidDataThreePrsntInt)
  [TrlrAidStsThreePrsntInt] -> CF100A_FordCanSigVldFlgGenr/24(TrlrAidStsThreePrsntInt)
  [FordVehTrsmDesGearRawVldInt] -> CF100A_FordCanSigVldFlgGenr/25(TrsmDesGearRawVldInt)
  CF100A_FordCanSigVldFlgGenr/1(FordVehActvFrntSteerModSteerWhlAg) -> [FordVehActvFrntSteerModlSteerWhlAgRawPassd]
  CF100A_FordCanSigVldFlgGenr/2(FordVehActvParkAssiVld) -> [FordVehActvParkAssiVld]
  CF100A_FordCanSigVldFlgGenr/3(FordVehGearLvrPosn) -> [FordVehGearLvrPosnPassd]
  CF100A_FordCanSigVldFlgGenr/4(FordVehGearLvrPosnVld) -> [FordVehGearLvrPosnVld]
  CF100A_FordCanSigVldFlgGenr/5(FordVehGearPosn) -> [FordVehGearPosnRawPassd]
  CF100A_FordCanSigVldFlgGenr/6(FordVehParkAidModlReqdAg) -> [FordVehParkAidModlReqdAgPassd]
  CF100A_FordCanSigVldFlgGenr/7(FordVehParkAidModlReqdSts) -> [FordVehParkAidModlReqdStsPassd]
  CF100A_FordCanSigVldFlgGenr/8(FordVehTrlrAgOffsDir) -> [FordVehTrlrAgOffsDirRawPassd]
  CF100A_FordCanSigVldFlgGenr/9(FordVehTrlrAidIdnNr) -> [FordVehTrlrAidIdnNrRawPassd]
  CF100A_FordCanSigVldFlgGenr/10(FordVehTrlrAidSetUp) -> [FordVehTrlrAidSetUpRawPassd]
  CF100A_FordCanSigVldFlgGenr/11(FordVehTrlrAidTrlrRvsGuidcSts) -> [FordVehTrlrAidTrlrRvsGuidcStsPassd]
  CF100A_FordCanSigVldFlgGenr/12(FordVehTrlrBackUpAssiEnaVld) -> [FordVehTrlrBackUpAssiEnaVld]
  CF100A_FordCanSigVldFlgGenr/13(FordVehTrlrBackUpAssiRvsVld) -> [FordVehTrlrBackUpAssiRvsVld]
  CF100A_FordCanSigVldFlgGenr/14(FordVehTrlrEnaReq) -> [FordVehTrlrEnaReqRawPassd]
  CF100A_FordCanSigVldFlgGenr/15(FordVehTrlrIdnTyp) -> [FordVehTrlrIdnTypRawPassd]
  CF100A_FordCanSigVldFlgGenr/16(FordVehTrlrRvsCnclReq) -> [FordVehTrlrRvsCnclReqRawPassd]
  CF100A_FordCanSigVldFlgGenr/17(FordVehTrlrRvsEna) -> [FordVehTrlrRvsEnaRawPassd]
  CF100A_FordCanSigVldFlgGenr/18(FordVehTrlrRvsMsgTxtReq) -> [FordVehTrlrRvsMsgTxtReqRawPassd]
  CF100A_FordCanSigVldFlgGenr/19(FordVehTrsmDesGear) -> [FordVehTrsmDesGearRawPassd]
